simulink model "simulink1"  (R2016a)
settings: Solver=VariableStepAuto  StartTime=0.0  StopTime=10.0  RelTol=1e-3
settings Model: Creator=hdt04  LastModifiedBy=hdt04

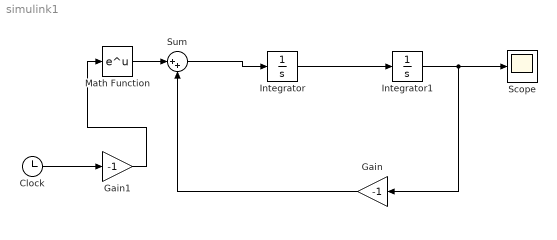
== system simulink1 ==
  Clock : Clock
  Gain : Gain  Gain=-1
  Gain1 : Gain  Gain=-1
  Integrator : Integrator
  Integrator1 : Integrator  InitialCondition=1
  Math Function : Math  SaturateOnIntegerOverflow=on
  Scope : Scope
  Sum : Sum  Inputs=|++
  wires:
  Integrator/1 -> Integrator1/1
  Integrator1/1 -> Gain/1, Scope/1
  Gain1/1 -> Math Function/1
  Clock/1 -> Gain1/1
  Gain/1 -> Sum/2
  Math Function/1 -> Sum/1
  Sum/1 -> Integrator/1
